simulink model "model"  (R2022a)
settings: Solver=VariableStepAuto  StartTime=0.0  StopTime=10.0  RelTol=1e-6
values from neighbouring files (symbols this model uses):
  K_oc = 1.2    [task1.m]
  K_oy = 9.8    [config.m]
  T = 0.2    [config.m]
settings Model: Creator=Vvlad  LastModifiedBy=Vvlad

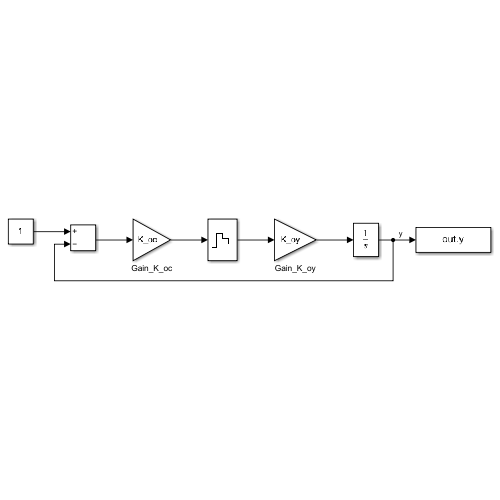
[thumbnail: Simulink's stored preview of the top-level diagram]
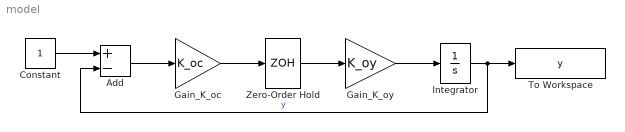
== system model ==
  Add : Sum  Inputs=+-
  Constant : Constant
  Gain_K_oc : Gain  Gain=K_oc
  Gain_K_oy : Gain  Gain=K_oy
  Integrator : Integrator
  To Workspace : ToWorkspace  VariableName=y  SampleTime=-1
  Zero-Order Hold : ZeroOrderHold  SampleTime=T
  wires:
  Add/1 -> Gain_K_oc/1
  Gain_K_oy/1 -> Integrator/1
  Integrator/1 -> To Workspace/1, Add/2  "y"
  Zero-Order Hold/1 -> Gain_K_oy/1
  Gain_K_oc/1 -> Zero-Order Hold/1
  Constant/1 -> Add/1
